simulink model "function_call_Subsystem"  (R2024a)
settings: Solver=FixedStepAuto  StartTime=0.0  StopTime=10.0  RelTol=1e-3
settings Model: Creator=DELL  LastModifiedBy=DELL
settings OptimizationCC: DefaultParameterBehavior=Inlined  EnhancedBackFolding=on  PassReuseOutputArgsAs=Individual arguments  ZeroExternalMemoryAtStartup=off  ZeroInternalMemoryAtStartup=off  OptimizeBlockOrder=speed  DifferentSizesBufferReuse=on  OptimizationCustomize=off  EfficientTunableParamExpr=on
settings DebuggingCC: ParameterTunabilityLossMsg=error
settings SFSimCC: MATLABDynamicMemAlloc=off
settings RTWCC: Description=Embedded Coder  SystemTargetFile=ert.tlc  TemplateMakefile=ert_default_tmf
settings CodeAppCC: ForceParamTrailComments=on  IgnoreCustomStorageClasses=off  OperatorAnnotations=on  SimulinkDataObjDesc=on  SFDataObjDesc=on  InsertBlockDesc=on
settings ERTTargetCC: TargetLangStandard=C99 (ISO)  GenerateSampleERTMain=on  InlinedParameterPlacement=NonHierarchical  ERTCustomFileTemplate=example_file_process.tlc

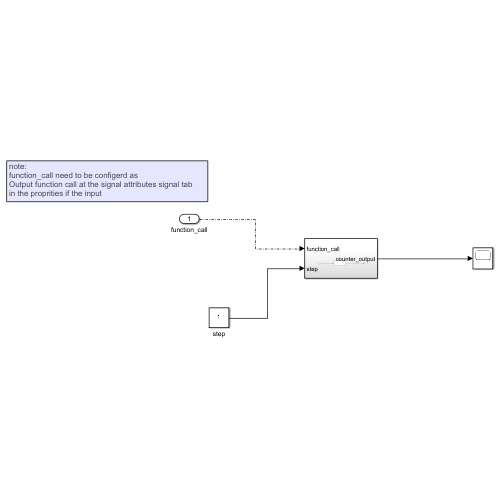
[thumbnail: Simulink's stored preview of the top-level diagram]
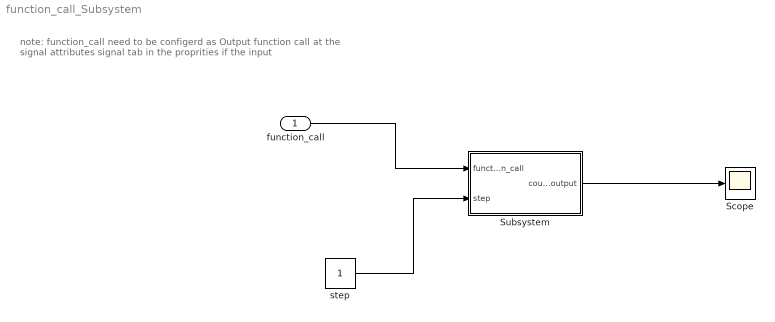
== system function_call_Subsystem ==
  note: note:
      | function_call need to be configerd as
      | Output function call at the signal attributes signal tab
      | in the proprities if the input
  function_call : Inport  OutputFunctionCall=on
  Scope : Scope
  Subsystem : Subsystem
  step : Constant
  wires:
  function_call/1 -> Subsystem/1(function_call)
  Subsystem/1(counter_output) -> Scope/1
  step/1 -> Subsystem/2(step)

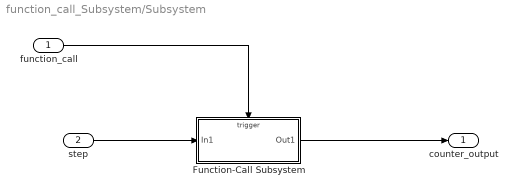
== system function_call_Subsystem/Subsystem ==
  function_call : Inport
  step : Inport  Port=2
  Function-Call Subsystem : Subsystem  TreatAsAtomicUnit=on
  counter_output : Outport
  wires:
  function_call/1 -> Function-Call Subsystem/Trigger
  step/1 -> Function-Call Subsystem/1(In1)
  Function-Call Subsystem/1(Out1) -> counter_output/1

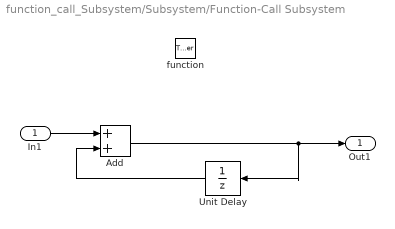
== system function_call_Subsystem/Subsystem/Function-Call Subsystem ==
  In1 : Inport
  function : TriggerPort  TriggerType=function-call  VariantControl=(inherit)
  Add : Sum
  Unit Delay : UnitDelay  SampleTime=-1  HasFrameUpgradeWarning=on
  Out1 : Outport
  wires:
  In1/1 -> Add/1
  Add/1 -> Unit Delay/1, Out1/1
  Unit Delay/1 -> Add/2
